simulink library "dynamics_lib"  (R2016b)
settings: Solver=ode45  StartTime=0.0  StopTime=10.0  RelTol=1e-3  EnableMultiTasking=on
undefined symbols (not defined in the file or in its folder): body_rates_radps, DiscIntNeverNeededParam, fsw_params, position_eci_km, quaternion, sim_params, velocity_eci_kmps
libraries: aerolibutil x6, vrlib x1, bus_stubs_template x1
settings Model: Creator=bbarz_000  LastModifiedBy=Taylor
settings DataIOCC: LimitDataPoints=on
settings OptimizationCC: LifeSpan=inf
settings DebuggingCC: AllowSymbolicDim=off  SFUnexpectedBacktrackingDiag=warning  SFNoUnconditionalDefaultTransitionDiag=warning  SFExecutionAtInitializationDiag=none
settings GRTTargetCC: TargetLangStandard=C89/C90 (ANSI)  GeneratePreprocessorConditionals=Disable all
settings ConfigComp: CovMetricSettings=dw  CovHtmlReporting=on  CovSaveCumulativeToWorkspaceVar=on  CovSaveSingleToWorkspaceVar=on  CovExternalEMLEnable=off

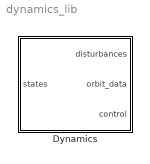
== system dynamics_lib ==
  Dynamics : Subsystem

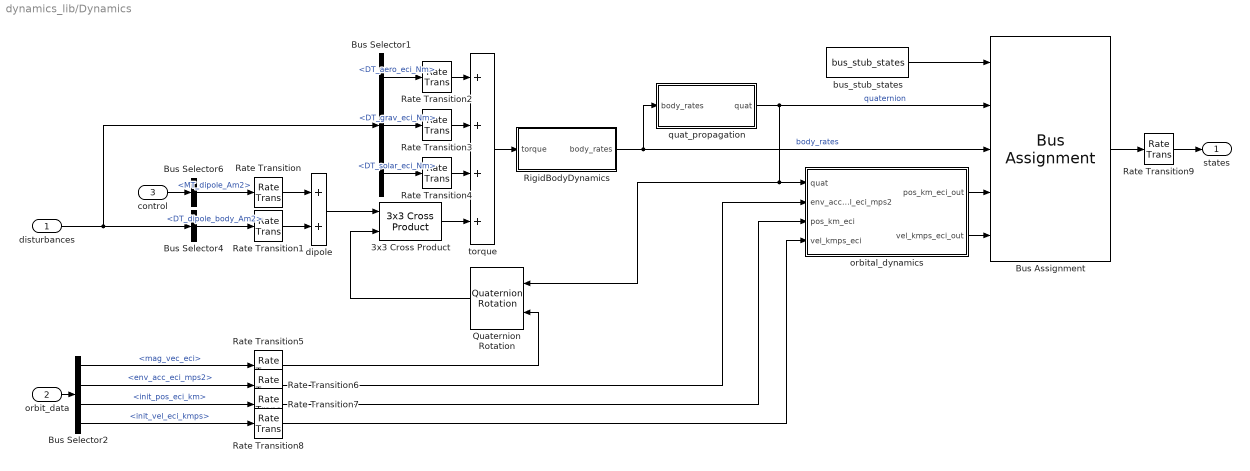
== system dynamics_lib/Dynamics ==
  disturbances : Inport  OutDataTypeStr=Bus: disturbances
  orbit_data : Inport  Port=2  OutDataTypeStr=Bus: orbit_data
  control : Inport  Port=3  OutDataTypeStr=Bus: control
  3x3 Cross Product : aerolibutil/3x3 Cross Product
  Bus Assignment : BusAssignment  AssignedSignals=quaternion,body_rates_radps,position_eci_km,velocity_eci_kmps
  Bus Selector1 : BusSelector  OutputSignals=DT_aero_eci_Nm,DT_grav_eci_Nm,DT_solar_eci_Nm
  Bus Selector2 : BusSelector  OutputSignals=mag_vec_eci,env_acc_eci_mps2,init_pos_eci_km,init_vel_eci_kmps
  Bus Selector4 : BusSelector  OutputSignals=DT_dipole_body_Am2
  Bus Selector6 : BusSelector  OutputSignals=MT_dipole_Am2
  Quaternion Rotation : aerolibutil/Quaternion Rotation
  Rate Transition{,1..6} (7 alike) : RateTransition  OutPortSampleTime=sim_params.sample_time_s
  Rate Transition7 : RateTransition  X0=fsw_params.constants.ic.pos_eci_m*1e-3  OutPortSampleTime=sim_params.sample_time_s
  Rate Transition8 : RateTransition  X0=fsw_params.constants.ic.vel_eci_mps * 1e-3  OutPortSampleTime=sim_params.sample_time_s
  Rate Transition9 : RateTransition
  RigidBodyDynamics : Subsystem
  bus_stub_states : bus_stubs_template/bus_stub_states
  dipole : Sum  Inputs=2
  orbital_dynamics : Subsystem
  quat_propagation : Subsystem
  torque : Sum  Inputs=4
  states : Outport
  wires:
  Bus Assignment/1 -> Rate Transition9/1
  bus_stub_states/1 -> Bus Assignment/1
  quat_propagation/1(quat) -> orbital_dynamics/1(quat), Quaternion Rotation/1, Bus Assignment/2  "quaternion"
  RigidBodyDynamics/1(body_rates) -> quat_propagation/1(body_rates), Bus Assignment/3  "body_rates"
  disturbances/1 -> Bus Selector1/1, Bus Selector4/1
  Bus Selector1/1 -> Rate Transition2/1  "<DT_aero_eci_Nm>"
  Bus Selector1/2 -> Rate Transition3/1  "<DT_grav_eci_Nm>"
  Bus Selector1/3 -> Rate Transition4/1  "<DT_solar_eci_Nm>"
  control/1 -> Bus Selector6/1
  Bus Selector4/1 -> Rate Transition1/1  "<DT_dipole_body_Am2>"
  Bus Selector6/1 -> Rate Transition/1  "<MT_dipole_Am2>"
  torque/1 -> RigidBodyDynamics/1(torque)
  dipole/1 -> 3x3 Cross Product/1
  Quaternion Rotation/1 -> 3x3 Cross Product/2
  3x3 Cross Product/1 -> torque/4
  Bus Selector2/2 -> Rate Transition6/1  "<env_acc_eci_mps2>"
  Bus Selector2/1 -> Rate Transition5/1  "<mag_vec_eci>"
  orbital_dynamics/2(vel_kmps_eci_out) -> Bus Assignment/5
  orbital_dynamics/1(pos_km_eci_out) -> Bus Assignment/4
  Bus Selector2/3 -> Rate Transition7/1  "<init_pos_eci_km>"
  Bus Selector2/4 -> Rate Transition8/1  "<init_vel_eci_kmps>"
  orbit_data/1 -> Bus Selector2/1
  Rate Transition/1 -> dipole/1
  Rate Transition1/1 -> dipole/2
  Rate Transition2/1 -> torque/1
  Rate Transition3/1 -> torque/2
  Rate Transition4/1 -> torque/3
  Rate Transition5/1 -> Quaternion Rotation/2
  Rate Transition6/1 -> orbital_dynamics/2(env_accel_eci_mps2)
  Rate Transition7/1 -> orbital_dynamics/3(pos_km_eci)
  Rate Transition8/1 -> orbital_dynamics/4(vel_kmps_eci)
  Rate Transition9/1 -> states/1

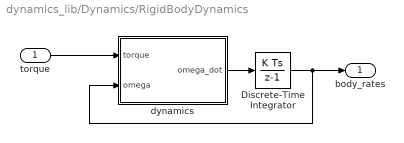
== system dynamics_lib/Dynamics/RigidBodyDynamics ==
  torque : Inport
  Discrete-Time Integrator : DiscreteIntegrator  InitialCondition=sim_params.dynamics.ic.rate_init  InitialConditionSetting=State (most efficient)  SampleTime=-1  ICPrevOutput=DiscIntNeverNeededParam  ICPrevScaledInput=DiscIntNeverNeededParam
  dynamics : Subsystem
  body_rates : Outport
  wires:
  dynamics/1(omega_dot) -> Discrete-Time Integrator/1
  torque/1 -> dynamics/1(torque)
  Discrete-Time Integrator/1 -> dynamics/2(omega), body_rates/1

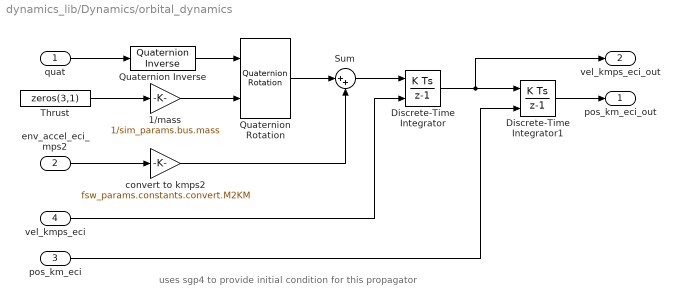
== system dynamics_lib/Dynamics/orbital_dynamics ==
  note: uses sgp4 to provide initial condition for this propagator
  quat : Inport
  env_accel_eci_mps2 : Inport  Port=2
  pos_km_eci : Inport  Port=3
  vel_kmps_eci : Inport  Port=4
  1/mass : Gain  Gain=1/sim_params.bus.mass
  Discrete-Time Integrator : DiscreteIntegrator  InitialConditionSource=external  InitialConditionSetting=State (most efficient)  SampleTime=-1  ICPrevOutput=DiscIntNeverNeededParam  ICPrevScaledInput=DiscIntNeverNeededParam
  Discrete-Time Integrator1 : DiscreteIntegrator  InitialConditionSource=external  InitialConditionSetting=State (most efficient)  SampleTime=-1  ICPrevOutput=DiscIntNeverNeededParam  ICPrevScaledInput=DiscIntNeverNeededParam
  Quaternion Inverse : aerolibutil/Quaternion Inverse
  Quaternion Rotation : aerolibutil/Quaternion Rotation
  Sum : Sum  Inputs=|++
  Thrust : Constant  Value=zeros(3,1)  SampleTime=sim_params.sample_time_s
  convert to kmps2 : Gain  Gain=fsw_params.constants.convert.M2KM
  pos_km_eci_out : Outport
  vel_kmps_eci_out : Outport  Port=2
  wires:
  convert to kmps2/1 -> Sum/2
  Quaternion Rotation/1 -> Sum/1
  vel_kmps_eci/1 -> Discrete-Time Integrator/2
  env_accel_eci_mps2/1 -> convert to kmps2/1
  Discrete-Time Integrator/1 -> Discrete-Time Integrator1/1, vel_kmps_eci_out/1
  Thrust/1 -> 1/mass/1
  Sum/1 -> Discrete-Time Integrator/1
  1/mass/1 -> Quaternion Rotation/2
  Quaternion Inverse/1 -> Quaternion Rotation/1
  pos_km_eci/1 -> Discrete-Time Integrator1/2
  quat/1 -> Quaternion Inverse/1
  Discrete-Time Integrator1/1 -> pos_km_eci_out/1

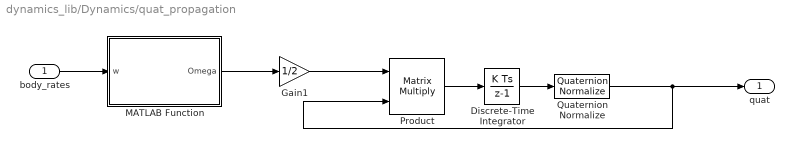
== system dynamics_lib/Dynamics/quat_propagation ==
  body_rates : Inport
  Discrete-Time Integrator : DiscreteIntegrator  InitialCondition=sim_params.dynamics.ic.quat_init  InitialConditionSetting=State (most efficient)  SampleTime=-1  ICPrevOutput=DiscIntNeverNeededParam  ICPrevScaledInput=DiscIntNeverNeededParam
  Gain1 : Gain  Gain=1/2
  MATLAB Function : MATLAB Function  TreatAsAtomicUnit=on
  Product : Product  Multiplication=Matrix(*)  RndMeth=Zero
  Quaternion Normalize : aerolibutil/Quaternion Normalize
  quat : Outport
  wires:
  MATLAB Function/1(Omega) -> Gain1/1
  body_rates/1 -> MATLAB Function/1(w)
  Quaternion Normalize/1 -> Product/2, quat/1
  Gain1/1 -> Product/1
  Discrete-Time Integrator/1 -> Quaternion Normalize/1
  Product/1 -> Discrete-Time Integrator/1

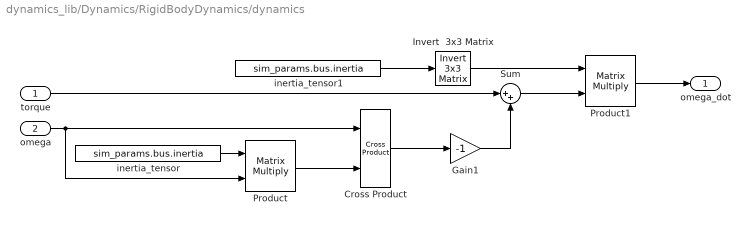
== system dynamics_lib/Dynamics/RigidBodyDynamics/dynamics ==
  torque : Inport
  omega : Inport  Port=2
  Cross Product : vrlib/Utilities/Cross Product
  Gain1 : Gain  Gain=-1
  Invert  3x3 Matrix : aerolibutil/Invert  3x3 Matrix
  Product : Product  Multiplication=Matrix(*)  RndMeth=Zero
  Product1 : Product  Multiplication=Matrix(*)  RndMeth=Zero
  Sum : Sum  Inputs=|++
  inertia_tensor : Constant  Value=sim_params.bus.inertia  SampleTime=sim_params.sample_time_s
  inertia_tensor1 : Constant  Value=sim_params.bus.inertia  SampleTime=sim_params.sample_time_s
  omega_dot : Outport
  wires:
  torque/1 -> Sum/1
  omega/1 -> Cross Product/1, Product/2
  inertia_tensor/1 -> Product/1
  Cross Product/1 -> Gain1/1
  Sum/1 -> Product1/2
  Product1/1 -> omega_dot/1
  Invert  3x3 Matrix/1 -> Product1/1
  inertia_tensor1/1 -> Invert  3x3 Matrix/1
  Gain1/1 -> Sum/2
  Product/1 -> Cross Product/2

== matlab function dynamics_lib/Dynamics/quat_propagation/MATLAB Function ==
  data: w input; Omega output
function Omega = skew_sym(w)
%#codegen

    w_skew = ...
        [0 w(3) -w(2);
        -w(3) 0 w(1);
        w(2) -w(1) 0];

    Omega = ...
        [0 -w';
        w w_skew];
